simulink model "bspline_polytraj_ex1"  (R2020a)
settings: Solver=FixedStepAuto  StartTime=0.0  StopTime=inf  FixedStep=1/60  RelTol=1e-3
values from neighbouring files (symbols this model uses):
  B = jacobian(simfonction, U )    [GetAuvSimAndJacobian.m]    (also in PlantUpdate.m = M(1:nx,nx+1:nx+nu); test_Dynamic_Matix.m = [zeros(7,8);Minv*Tm])
undefined symbols (not defined in the file or in its folder): DiscIntNeverNeededParam, eul2tform, Spline, trvec2tform, waypoints
libraries: robotcorelib x4, simulink x2
settings Model: EnablePacing=on  Creator=The MathWorks, Inc.  LastModifiedBy=lamarre
settings SFSimCC: CustomCodeUndefinedFunction=UseInterfaceOnly

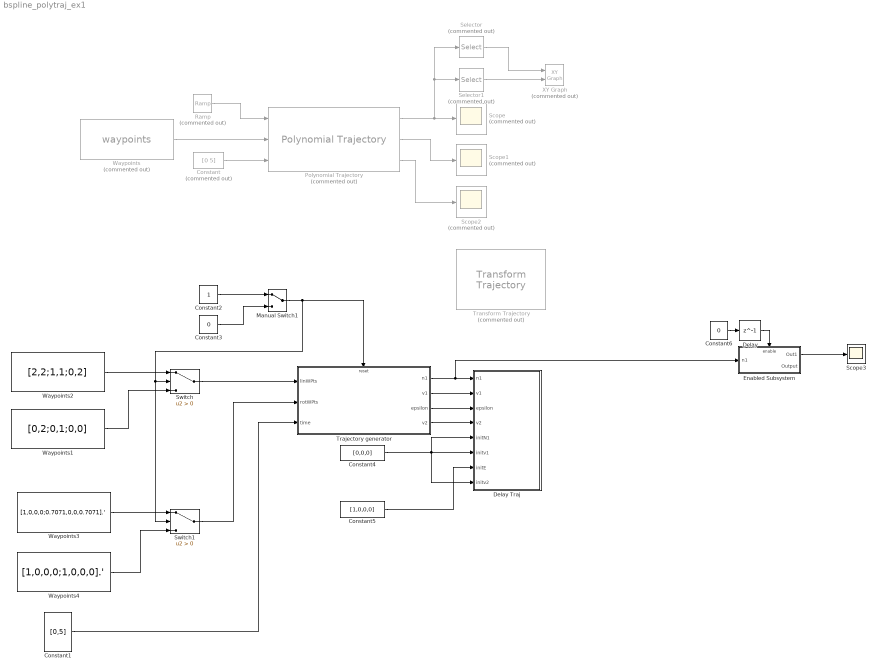
== system bspline_polytraj_ex1 ==
  Constant : Constant  Commented=on  Value=[0 5]
  Constant1 : Constant  Value=[0,5]  VectorParams1D=off
  Constant2 : Constant
  Constant3 : Constant  Value=0
  Constant4 : Constant  Value=[0,0,0]
  Constant5 : Constant  Value=[1,0,0,0]
  Constant6 : Constant  Value=0
  Delay : Delay  DelayLength=1  InitialCondition=1
  Delay Traj : Subsystem
  Enabled Subsystem : Subsystem  TreatAsAtomicUnit=on
  Manual Switch1 : ManualSwitch
  Polynomial Trajectory : robotcorelib/Polynomial Trajectory  Commented=on  WaypointSource=External  Waypoints=wayPoints  TimePoints=[ 0, 1, 2, 3, 4 ]  TimeInterval=[0,5]  Method=B-Spline  ParameterSource=Internal  VelocityBoundaryCondition=zeros( 2, 5 )  AccelerationBoundaryCondition=zeros( 2, 5 )  SimulateUsing=Interpreted execution
      settings: SourceProductBaseCode=NV,RO,RR
  Ramp : simulink/Sources/Ramp  Commented=on  slope=1  start=0  InitialOutput=0
  Scope : Scope  Commented=on
  Scope1 : Scope  Commented=on
  Scope2 : Scope  Commented=on
  Scope3 : Scope
  Selector : Selector  Commented=on  InputPortWidth=2  IndexOptions=Index vector (dialog)  Indices=1  OutputSizes=1
  Selector1 : Selector  Commented=on  InputPortWidth=2  IndexOptions=Index vector (dialog)  Indices=2  OutputSizes=1
  Switch : Switch  Criteria=u2 > Threshold
  Switch1 : Switch  Criteria=u2 > Threshold
  Trajectory generator : Subsystem
  Transform Trajectory : robotcorelib/Transform Trajectory  Commented=on  WaypointSource=Internal  T0=trvec2tform( [ 1, 10, -1 ] )  TF=eul2tform( [ 0, pi, pi / 2 ] )  TimeInterval=[ 2, 3 ]  CustomTimeScaling=off  ParameterSource=Internal  TSTime=2:0.1:3  TimeScaling=[ 0:0.1:1; ones( 1, 11 ); zeros( 1, 11 ) ]  SimulateUsing=Interpreted execution
      settings: SourceProductBaseCode=NV,RO,RR
  Waypoints : Constant  Commented=on  Value=waypoints
  Waypoints1 : Constant  Value=[0,2;0,1;0,0]
  Waypoints2 : Constant  Value=[2,2;1,1;0,2]
  Waypoints3 : Constant  Value=[1,0,0,0;0.7071,0,0,0.7071].'
  Waypoints4 : Constant  Value=[1,0,0,0;1,0,0,0].'
  XY Graph : simulink/Sinks/XY Graph  Commented=on  xmin=-3  xmax=5  ymin=-1  ymax=5  st=-1
  wires:
  Ramp/1 -> Polynomial Trajectory/1
  Polynomial Trajectory/1 -> Selector1/1, Selector/1, Scope/1
  Polynomial Trajectory/2 -> Scope1/1
  Polynomial Trajectory/3 -> Scope2/1
  Selector1/1 -> XY Graph/2
  Selector/1 -> XY Graph/1
  Constant/1 -> Polynomial Trajectory/3
  Waypoints/1 -> Polynomial Trajectory/2
  Constant1/1 -> Trajectory generator/3(time)
  Constant2/1 -> Manual Switch1/1
  Constant3/1 -> Manual Switch1/2
  Switch/1 -> Trajectory generator/1(linWPts)
  Waypoints1/1 -> Switch/3
  Waypoints2/1 -> Switch/1
  Trajectory generator/1(n1) -> Enabled Subsystem/1(n1), Delay Traj/1(n1)
  Manual Switch1/1 -> Switch/2, Switch1/2, Trajectory generator/Reset
  Waypoints3/1 -> Switch1/1
  Waypoints4/1 -> Switch1/3
  Switch1/1 -> Trajectory generator/2(rotWPts)
  Trajectory generator/2(v1) -> Delay Traj/2(v1)
  Trajectory generator/3(epsilon) -> Delay Traj/3(epsilon)
  Trajectory generator/4(v2) -> Delay Traj/4(v2)
  Constant4/1 -> Delay Traj/8(initv2), Delay Traj/6(initv1), Delay Traj/5(initN1)
  Constant5/1 -> Delay Traj/7(initE)
  Delay/1 -> Enabled Subsystem/Enable
  Enabled Subsystem/1(Out1) -> Scope3/1
  Constant6/1 -> Delay/1

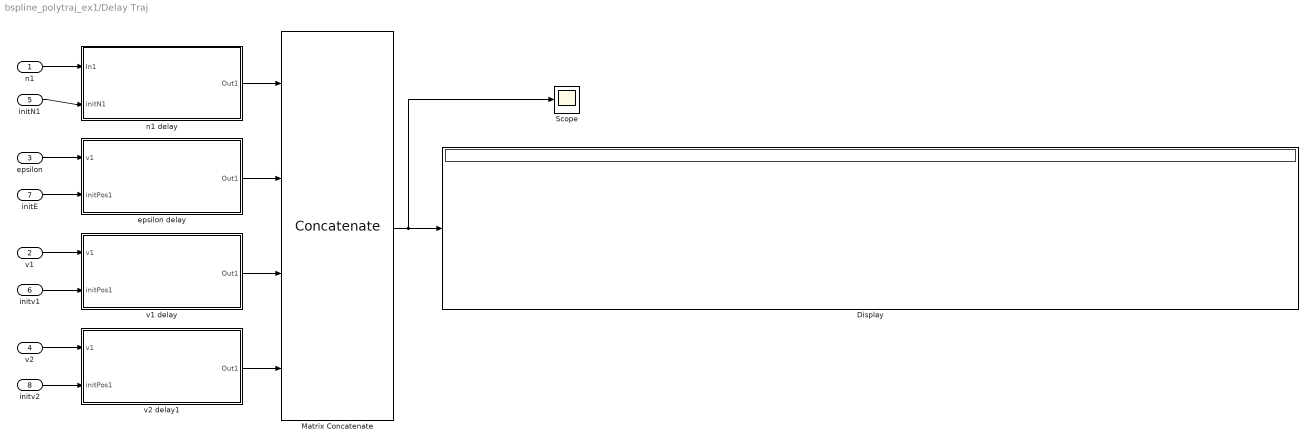
== system bspline_polytraj_ex1/Delay Traj ==
  n1 : Inport
  v1 : Inport  Port=2
  epsilon : Inport  Port=3
  v2 : Inport  Port=4
  initN1 : Inport  Port=5
  initv1 : Inport  Port=6
  initE : Inport  Port=7
  initv2 : Inport  Port=8
  Display : Display
  Matrix Concatenate : Concatenate  NumInputs=4  Mode=Multidimensional array  ConcatenateDimension=2
  Scope : Scope
  epsilon delay : Subsystem
  n1 delay : Subsystem
  v1 delay : Subsystem
  v2 delay1 : Subsystem
  wires:
  n1/1 -> n1 delay/1(In1)
  n1 delay/1(Out1) -> Matrix Concatenate/1
  v1/1 -> v1 delay/1(v1)
  epsilon/1 -> epsilon delay/1(v1)
  initN1/1 -> n1 delay/2(initN1)
  initv1/1 -> v1 delay/2(initPos1)
  initE/1 -> epsilon delay/2(initPos1)
  v2/1 -> v2 delay1/1(v1)
  initv2/1 -> v2 delay1/2(initPos1)
  v2 delay1/1(Out1) -> Matrix Concatenate/4
  Matrix Concatenate/1 -> Scope/1, Display/1
  v1 delay/1(Out1) -> Matrix Concatenate/3
  epsilon delay/1(Out1) -> Matrix Concatenate/2

== system bspline_polytraj_ex1/Enabled Subsystem ==
  n1 : Inport
  Enable : EnablePort
  Constant : Constant
  Out1 : Outport
  Output : Outport  Port=2
  wires:
  n1/1 -> Out1/1
  Constant/1 -> Output/1

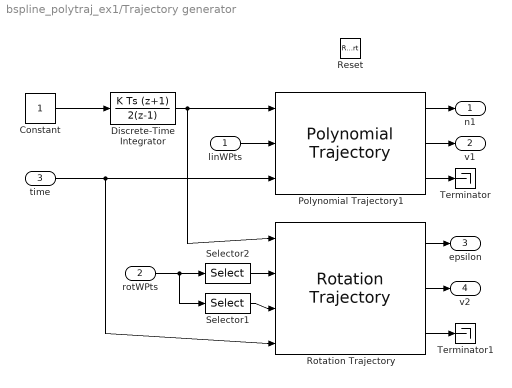
== system bspline_polytraj_ex1/Trajectory generator ==
  linWPts : Inport
  rotWPts : Inport  Port=2
  time : Inport  Port=3
  Reset : ResetPort  DisableCoverage=on
  Constant : Constant
  Discrete-Time Integrator : DiscreteIntegrator  IntegratorMethod=Integration: Trapezoidal  SampleTime=.25  ICPrevOutput=DiscIntNeverNeededParam  ICPrevScaledInput=DiscIntNeverNeededParam
  Polynomial Trajectory1 : robotcorelib/Polynomial Trajectory  WaypointSource=External  Waypoints=wayPoints  TimePoints=[ 0, 1, 2, 3, 4 ]  TimeInterval=[0,5]  Method=Cubic Polynomial  ParameterSource=Internal  VelocityBoundaryCondition=zeros( 3, 2 )  AccelerationBoundaryCondition=zeros( 2, 5 )  SimulateUsing=Code generation
      settings: SourceProductBaseCode=NV,RO,RR
  Rotation Trajectory : robotcorelib/Rotation Trajectory  WaypointFormat=Quaternion  WaypointSource=External  R0=[ 1, 0, 0, 0 ]'  RF=[ 0, 0, 1, 0 ]'  TimeInterval=[ 0, 1 ]  CustomTimeScaling=off  ParameterSource=Internal  TSTime=0:0.1:1  TimeScaling=[ 0:0.1:1; ones( 1, 11 ); zeros( 1, 11 ) ]  SimulateUsing=Code generation
      settings: SourceProductBaseCode=NV,RO,RR
  Selector1 : Selector  NumberOfDimensions=2  InputPortWidth=3  IndexOptions=Index vector (dialog),Index vector (dialog)  Indices=[1:4],2  OutputSizes=1,1
  Selector2 : Selector  NumberOfDimensions=2  InputPortWidth=3  IndexOptions=Index vector (dialog),Index vector (dialog)  Indices=[1:4],1  OutputSizes=1,1
  Terminator : Terminator
  Terminator1 : Terminator
  n1 : Outport
  v1 : Outport  Port=2
  epsilon : Outport  Port=3
  v2 : Outport  Port=4
  wires:
  Polynomial Trajectory1/2 -> v1/1
  Polynomial Trajectory1/1 -> n1/1
  Polynomial Trajectory1/3 -> Terminator/1
  Constant/1 -> Discrete-Time Integrator/1
  Discrete-Time Integrator/1 -> Polynomial Trajectory1/1, Rotation Trajectory/1
  linWPts/1 -> Polynomial Trajectory1/2
  time/1 -> Rotation Trajectory/4, Polynomial Trajectory1/3
  Rotation Trajectory/2 -> v2/1
  Rotation Trajectory/1 -> epsilon/1
  Rotation Trajectory/3 -> Terminator1/1
  rotWPts/1 -> Selector1/1, Selector2/1
  Selector2/1 -> Rotation Trajectory/2
  Selector1/1 -> Rotation Trajectory/3

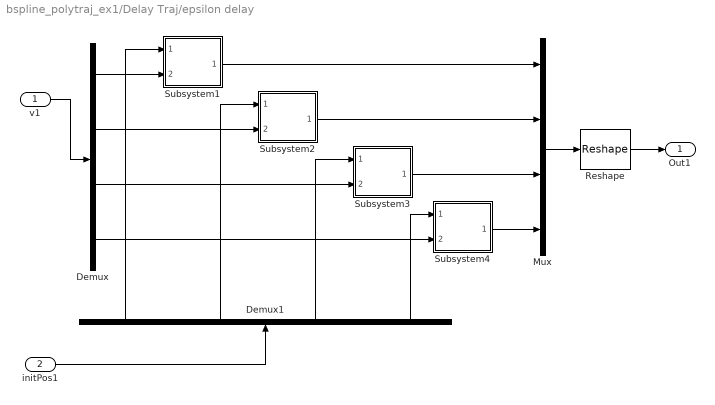
== system bspline_polytraj_ex1/Delay Traj/epsilon delay ==
  v1 : Inport
  initPos1 : Inport  Port=2
  Demux : Demux
  Demux1 : Demux
  Mux : Mux
  Reshape : Reshape  OutputDimensionality=Customize  OutputDimensions=[4,4]
  Subsystem1 : Subsystem
  Subsystem2 : Subsystem
  Subsystem3 : Subsystem
  Subsystem4 : Subsystem
  Out1 : Outport
  wires:
  Subsystem3/1(Out1) -> Mux/3
  Demux1/3 -> Subsystem3/1(Initcond)
  Demux1/1 -> Subsystem1/1(Initcond)
  Demux/1 -> Subsystem1/2(Signal)
  Mux/1 -> Reshape/1
  v1/1 -> Demux/1
  Demux1/2 -> Subsystem2/1(Initcond)
  Subsystem2/1(Out1) -> Mux/2
  Subsystem1/1(Out1) -> Mux/1
  initPos1/1 -> Demux1/1
  Demux/3 -> Subsystem3/2(Signal)
  Reshape/1 -> Out1/1
  Demux/2 -> Subsystem2/2(Signal)
  Demux/4 -> Subsystem4/2(Signal)
  Subsystem4/1(Out1) -> Mux/4
  Demux1/4 -> Subsystem4/1(Initcond)

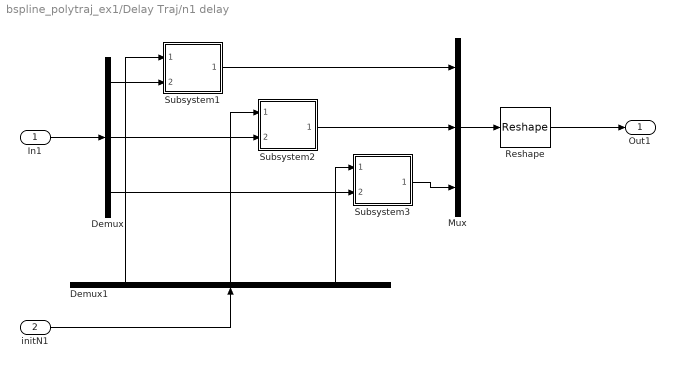
== system bspline_polytraj_ex1/Delay Traj/n1 delay ==
  In1 : Inport
  initN1 : Inport  Port=2
  Demux : Demux  Outputs=3
  Demux1 : Demux  Outputs=3
  Mux : Mux  Inputs=3
  Reshape : Reshape  OutputDimensionality=Customize  OutputDimensions=[4,3]
  Subsystem1 : Subsystem
  Subsystem2 : Subsystem
  Subsystem3 : Subsystem
  Out1 : Outport
  wires:
  Subsystem3/1(Out1) -> Mux/3
  Demux1/3 -> Subsystem3/1(Initcond)
  Demux1/1 -> Subsystem1/1(Initcond)
  Demux/1 -> Subsystem1/2(Signal)
  Mux/1 -> Reshape/1
  In1/1 -> Demux/1
  Demux1/2 -> Subsystem2/1(Initcond)
  Subsystem2/1(Out1) -> Mux/2
  Subsystem1/1(Out1) -> Mux/1
  initN1/1 -> Demux1/1
  Demux/3 -> Subsystem3/2(Signal)
  Reshape/1 -> Out1/1
  Demux/2 -> Subsystem2/2(Signal)

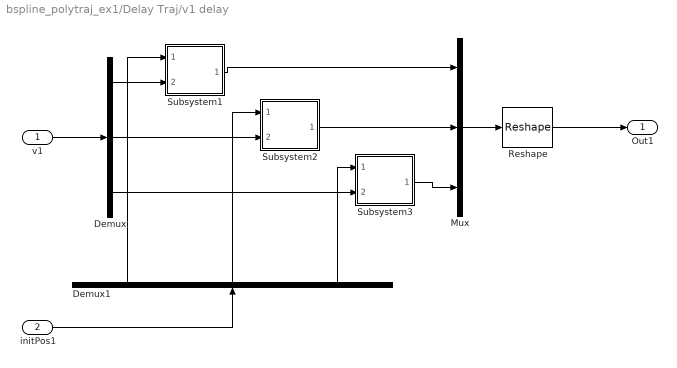
== system bspline_polytraj_ex1/Delay Traj/v1 delay ==
  v1 : Inport
  initPos1 : Inport  Port=2
  Demux : Demux  Outputs=3
  Demux1 : Demux  Outputs=3
  Mux : Mux  Inputs=3
  Reshape : Reshape  OutputDimensionality=Customize  OutputDimensions=[4,3]
  Subsystem1 : Subsystem
  Subsystem2 : Subsystem
  Subsystem3 : Subsystem
  Out1 : Outport
  wires:
  Subsystem3/1(Out1) -> Mux/3
  Demux1/3 -> Subsystem3/1(Initcond)
  Demux1/1 -> Subsystem1/1(Initcond)
  Demux/1 -> Subsystem1/2(Signal)
  Mux/1 -> Reshape/1
  v1/1 -> Demux/1
  Demux1/2 -> Subsystem2/1(Initcond)
  Subsystem2/1(Out1) -> Mux/2
  Subsystem1/1(Out1) -> Mux/1
  initPos1/1 -> Demux1/1
  Demux/3 -> Subsystem3/2(Signal)
  Reshape/1 -> Out1/1
  Demux/2 -> Subsystem2/2(Signal)

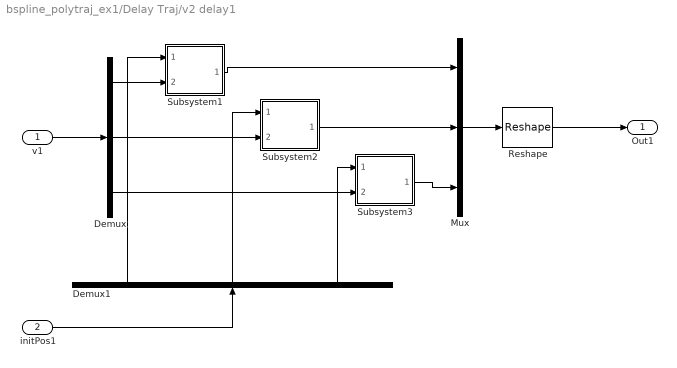
== system bspline_polytraj_ex1/Delay Traj/v2 delay1 ==
  v1 : Inport
  initPos1 : Inport  Port=2
  Demux : Demux  Outputs=3
  Demux1 : Demux  Outputs=3
  Mux : Mux  Inputs=3
  Reshape : Reshape  OutputDimensionality=Customize  OutputDimensions=[4,3]
  Subsystem1 : Subsystem
  Subsystem2 : Subsystem
  Subsystem3 : Subsystem
  Out1 : Outport
  wires:
  Subsystem3/1(Out1) -> Mux/3
  Demux1/3 -> Subsystem3/1(Initcond)
  Demux1/1 -> Subsystem1/1(Initcond)
  Demux/1 -> Subsystem1/2(Signal)
  Mux/1 -> Reshape/1
  v1/1 -> Demux/1
  Demux1/2 -> Subsystem2/1(Initcond)
  Subsystem2/1(Out1) -> Mux/2
  Subsystem1/1(Out1) -> Mux/1
  initPos1/1 -> Demux1/1
  Demux/3 -> Subsystem3/2(Signal)
  Reshape/1 -> Out1/1
  Demux/2 -> Subsystem2/2(Signal)

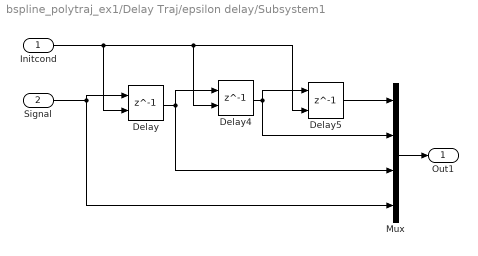
== system bspline_polytraj_ex1/Delay Traj/epsilon delay/Subsystem1 ==
  Initcond : Inport
  Signal : Inport  Port=2
  Delay : Delay  DelayLength=1  InitialConditionSource=Input port  InitialCondition=[0,0,0].'
      settings: InputPortMap=u0,p4
  Delay4 : Delay  DelayLength=1  InitialConditionSource=Input port  InitialCondition=[0,0,0].'
      settings: InputPortMap=u0,p4
  Delay5 : Delay  DelayLength=1  InitialConditionSource=Input port  InitialCondition=[0,0,0].'
      settings: InputPortMap=u0,p4
  Mux : Mux
  Out1 : Outport
  wires:
  Delay5/1 -> Mux/1
  Mux/1 -> Out1/1
  Signal/1 -> Delay/1, Mux/4
  Delay4/1 -> Mux/2, Delay5/1
  Delay/1 -> Delay4/1, Mux/3
  Initcond/1 -> Delay/2, Delay4/2, Delay5/2

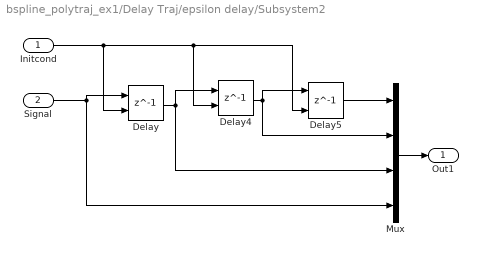
== system bspline_polytraj_ex1/Delay Traj/epsilon delay/Subsystem2 ==
  Initcond : Inport
  Signal : Inport  Port=2
  Delay : Delay  DelayLength=1  InitialConditionSource=Input port  InitialCondition=[0,0,0].'
      settings: InputPortMap=u0,p4
  Delay4 : Delay  DelayLength=1  InitialConditionSource=Input port  InitialCondition=[0,0,0].'
      settings: InputPortMap=u0,p4
  Delay5 : Delay  DelayLength=1  InitialConditionSource=Input port  InitialCondition=[0,0,0].'
      settings: InputPortMap=u0,p4
  Mux : Mux
  Out1 : Outport
  wires:
  Delay5/1 -> Mux/1
  Mux/1 -> Out1/1
  Signal/1 -> Delay/1, Mux/4
  Delay4/1 -> Mux/2, Delay5/1
  Delay/1 -> Delay4/1, Mux/3
  Initcond/1 -> Delay/2, Delay4/2, Delay5/2

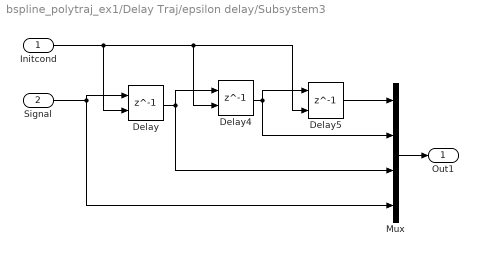
== system bspline_polytraj_ex1/Delay Traj/epsilon delay/Subsystem3 ==
  Initcond : Inport
  Signal : Inport  Port=2
  Delay : Delay  DelayLength=1  InitialConditionSource=Input port  InitialCondition=[0,0,0].'
      settings: InputPortMap=u0,p4
  Delay4 : Delay  DelayLength=1  InitialConditionSource=Input port  InitialCondition=[0,0,0].'
      settings: InputPortMap=u0,p4
  Delay5 : Delay  DelayLength=1  InitialConditionSource=Input port  InitialCondition=[0,0,0].'
      settings: InputPortMap=u0,p4
  Mux : Mux
  Out1 : Outport
  wires:
  Delay5/1 -> Mux/1
  Mux/1 -> Out1/1
  Signal/1 -> Delay/1, Mux/4
  Delay4/1 -> Mux/2, Delay5/1
  Delay/1 -> Delay4/1, Mux/3
  Initcond/1 -> Delay/2, Delay4/2, Delay5/2

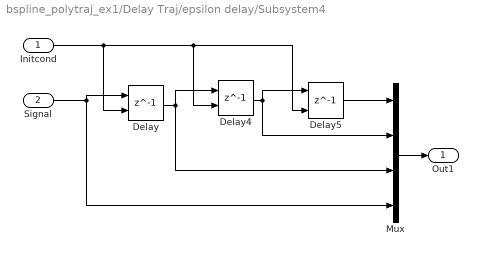
== system bspline_polytraj_ex1/Delay Traj/epsilon delay/Subsystem4 ==
  Initcond : Inport
  Signal : Inport  Port=2
  Delay : Delay  DelayLength=1  InitialConditionSource=Input port  InitialCondition=[0,0,0].'
      settings: InputPortMap=u0,p4
  Delay4 : Delay  DelayLength=1  InitialConditionSource=Input port  InitialCondition=[0,0,0].'
      settings: InputPortMap=u0,p4
  Delay5 : Delay  DelayLength=1  InitialConditionSource=Input port  InitialCondition=[0,0,0].'
      settings: InputPortMap=u0,p4
  Mux : Mux
  Out1 : Outport
  wires:
  Delay5/1 -> Mux/1
  Mux/1 -> Out1/1
  Signal/1 -> Delay/1, Mux/4
  Delay4/1 -> Mux/2, Delay5/1
  Delay/1 -> Delay4/1, Mux/3
  Initcond/1 -> Delay/2, Delay4/2, Delay5/2

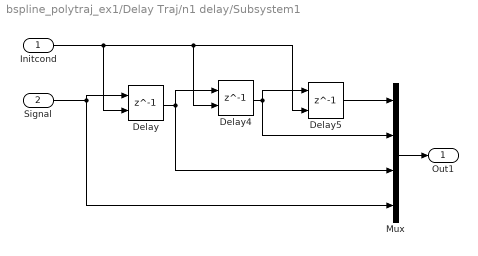
== system bspline_polytraj_ex1/Delay Traj/n1 delay/Subsystem1 ==
  Initcond : Inport
  Signal : Inport  Port=2
  Delay : Delay  DelayLength=1  InitialConditionSource=Input port  InitialCondition=[0,0,0].'
      settings: InputPortMap=u0,p4
  Delay4 : Delay  DelayLength=1  InitialConditionSource=Input port  InitialCondition=[0,0,0].'
      settings: InputPortMap=u0,p4
  Delay5 : Delay  DelayLength=1  InitialConditionSource=Input port  InitialCondition=[0,0,0].'
      settings: InputPortMap=u0,p4
  Mux : Mux
  Out1 : Outport
  wires:
  Delay5/1 -> Mux/1
  Mux/1 -> Out1/1
  Signal/1 -> Delay/1, Mux/4
  Delay4/1 -> Mux/2, Delay5/1
  Delay/1 -> Delay4/1, Mux/3
  Initcond/1 -> Delay/2, Delay4/2, Delay5/2

== system bspline_polytraj_ex1/Delay Traj/n1 delay/Subsystem2 ==
  Initcond : Inport
  Signal : Inport  Port=2
  Delay : Delay  DelayLength=1  InitialConditionSource=Input port  InitialCondition=[0,0,0].'
      settings: InputPortMap=u0,p4
  Delay4 : Delay  DelayLength=1  InitialConditionSource=Input port  InitialCondition=[0,0,0].'
      settings: InputPortMap=u0,p4
  Delay5 : Delay  DelayLength=1  InitialConditionSource=Input port  InitialCondition=[0,0,0].'
      settings: InputPortMap=u0,p4
  Mux : Mux
  Out1 : Outport
  wires:
  Delay5/1 -> Mux/1
  Mux/1 -> Out1/1
  Signal/1 -> Delay/1, Mux/4
  Delay4/1 -> Mux/2, Delay5/1
  Delay/1 -> Delay4/1, Mux/3
  Initcond/1 -> Delay/2, Delay4/2, Delay5/2

== system bspline_polytraj_ex1/Delay Traj/n1 delay/Subsystem3 ==
  Initcond : Inport
  Signal : Inport  Port=2
  Delay : Delay  DelayLength=1  InitialConditionSource=Input port  InitialCondition=[0,0,0].'
      settings: InputPortMap=u0,p4
  Delay4 : Delay  DelayLength=1  InitialConditionSource=Input port  InitialCondition=[0,0,0].'
      settings: InputPortMap=u0,p4
  Delay5 : Delay  DelayLength=1  InitialConditionSource=Input port  InitialCondition=[0,0,0].'
      settings: InputPortMap=u0,p4
  Mux : Mux
  Out1 : Outport
  wires:
  Delay5/1 -> Mux/1
  Mux/1 -> Out1/1
  Signal/1 -> Delay/1, Mux/4
  Delay4/1 -> Mux/2, Delay5/1
  Delay/1 -> Delay4/1, Mux/3
  Initcond/1 -> Delay/2, Delay4/2, Delay5/2

== system bspline_polytraj_ex1/Delay Traj/v1 delay/Subsystem1 ==
  Initcond : Inport
  Signal : Inport  Port=2
  Delay : Delay  DelayLength=1  InitialConditionSource=Input port  InitialCondition=[0,0,0].'
      settings: InputPortMap=u0,p4
  Delay4 : Delay  DelayLength=1  InitialConditionSource=Input port  InitialCondition=[0,0,0].'
      settings: InputPortMap=u0,p4
  Delay5 : Delay  DelayLength=1  InitialConditionSource=Input port  InitialCondition=[0,0,0].'
      settings: InputPortMap=u0,p4
  Mux : Mux
  Out1 : Outport
  wires:
  Delay5/1 -> Mux/1
  Mux/1 -> Out1/1
  Signal/1 -> Delay/1, Mux/4
  Delay4/1 -> Mux/2, Delay5/1
  Delay/1 -> Delay4/1, Mux/3
  Initcond/1 -> Delay/2, Delay4/2, Delay5/2

== system bspline_polytraj_ex1/Delay Traj/v1 delay/Subsystem2 ==
  Initcond : Inport
  Signal : Inport  Port=2
  Delay : Delay  DelayLength=1  InitialConditionSource=Input port  InitialCondition=[0,0,0].'
      settings: InputPortMap=u0,p4
  Delay4 : Delay  DelayLength=1  InitialConditionSource=Input port  InitialCondition=[0,0,0].'
      settings: InputPortMap=u0,p4
  Delay5 : Delay  DelayLength=1  InitialConditionSource=Input port  InitialCondition=[0,0,0].'
      settings: InputPortMap=u0,p4
  Mux : Mux
  Out1 : Outport
  wires:
  Delay5/1 -> Mux/1
  Mux/1 -> Out1/1
  Signal/1 -> Delay/1, Mux/4
  Delay4/1 -> Mux/2, Delay5/1
  Delay/1 -> Delay4/1, Mux/3
  Initcond/1 -> Delay/2, Delay4/2, Delay5/2

== system bspline_polytraj_ex1/Delay Traj/v1 delay/Subsystem3 ==
  Initcond : Inport
  Signal : Inport  Port=2
  Delay : Delay  DelayLength=1  InitialConditionSource=Input port  InitialCondition=[0,0,0].'
      settings: InputPortMap=u0,p4
  Delay4 : Delay  DelayLength=1  InitialConditionSource=Input port  InitialCondition=[0,0,0].'
      settings: InputPortMap=u0,p4
  Delay5 : Delay  DelayLength=1  InitialConditionSource=Input port  InitialCondition=[0,0,0].'
      settings: InputPortMap=u0,p4
  Mux : Mux
  Out1 : Outport
  wires:
  Delay5/1 -> Mux/1
  Mux/1 -> Out1/1
  Signal/1 -> Delay/1, Mux/4
  Delay4/1 -> Mux/2, Delay5/1
  Delay/1 -> Delay4/1, Mux/3
  Initcond/1 -> Delay/2, Delay4/2, Delay5/2

== system bspline_polytraj_ex1/Delay Traj/v2 delay1/Subsystem1 ==
  Initcond : Inport
  Signal : Inport  Port=2
  Delay : Delay  DelayLength=1  InitialConditionSource=Input port  InitialCondition=[0,0,0].'
      settings: InputPortMap=u0,p4
  Delay4 : Delay  DelayLength=1  InitialConditionSource=Input port  InitialCondition=[0,0,0].'
      settings: InputPortMap=u0,p4
  Delay5 : Delay  DelayLength=1  InitialConditionSource=Input port  InitialCondition=[0,0,0].'
      settings: InputPortMap=u0,p4
  Mux : Mux
  Out1 : Outport
  wires:
  Delay5/1 -> Mux/1
  Mux/1 -> Out1/1
  Signal/1 -> Delay/1, Mux/4
  Delay4/1 -> Mux/2, Delay5/1
  Delay/1 -> Delay4/1, Mux/3
  Initcond/1 -> Delay/2, Delay4/2, Delay5/2

== system bspline_polytraj_ex1/Delay Traj/v2 delay1/Subsystem2 ==
  Initcond : Inport
  Signal : Inport  Port=2
  Delay : Delay  DelayLength=1  InitialConditionSource=Input port  InitialCondition=[0,0,0].'
      settings: InputPortMap=u0,p4
  Delay4 : Delay  DelayLength=1  InitialConditionSource=Input port  InitialCondition=[0,0,0].'
      settings: InputPortMap=u0,p4
  Delay5 : Delay  DelayLength=1  InitialConditionSource=Input port  InitialCondition=[0,0,0].'
      settings: InputPortMap=u0,p4
  Mux : Mux
  Out1 : Outport
  wires:
  Delay5/1 -> Mux/1
  Mux/1 -> Out1/1
  Signal/1 -> Delay/1, Mux/4
  Delay4/1 -> Mux/2, Delay5/1
  Delay/1 -> Delay4/1, Mux/3
  Initcond/1 -> Delay/2, Delay4/2, Delay5/2

== system bspline_polytraj_ex1/Delay Traj/v2 delay1/Subsystem3 ==
  Initcond : Inport
  Signal : Inport  Port=2
  Delay : Delay  DelayLength=1  InitialConditionSource=Input port  InitialCondition=[0,0,0].'
      settings: InputPortMap=u0,p4
  Delay4 : Delay  DelayLength=1  InitialConditionSource=Input port  InitialCondition=[0,0,0].'
      settings: InputPortMap=u0,p4
  Delay5 : Delay  DelayLength=1  InitialConditionSource=Input port  InitialCondition=[0,0,0].'
      settings: InputPortMap=u0,p4
  Mux : Mux
  Out1 : Outport
  wires:
  Delay5/1 -> Mux/1
  Mux/1 -> Out1/1
  Signal/1 -> Delay/1, Mux/4
  Delay4/1 -> Mux/2, Delay5/1
  Delay/1 -> Delay4/1, Mux/3
  Initcond/1 -> Delay/2, Delay4/2, Delay5/2
